simulink model "actuator_control"  (R2016b)
settings: configuration reference "Configuration4khz" (kept outside this file)
values from neighbouring files (symbols this model uses):
  sample_time = 0.0005    [ElmoIncremental.m]
undefined symbols (not defined in the file or in its folder): A_kalman_sea_swing_back, A_kalman_sea_swing_front, A_kalman_swing_load, A_lpf_1to4, A_lpf_dtau, A_lpf_sea_kalman_velocities, B1_lpf_1to4, B1_lpf_dtau, B1_lpf_sea_kalman_velocities, B2_lpf_1to4, B2_lpf_dtau, B2_lpf_sea_kalman_velocities, B_kalman_sea_swing_back, B_kalman_sea_swing_front, B_kalman_swing_load, C_kalman_sea_swing, C_kalman_swing_load, DiscIntNeverNeededParam, Discrete, elmo_sample_time, fdesignblkfcn, gcbh, initial_dx_estimate, j_segments, k_sea_low, kalman_load_to_deflect_transmission, lateral_motor_efficiency, LEG_MTR_GEAR_RATIO, P0_kalman_sea_swing, P0_kalman_swing_load, Q_kalman_load_torque, Q_kalman_rotor_torque, Q_kalman_trunk_torque, R_kalman_absolute_fail, R_kalman_absolute_normal, R_kalman_incremental_loaded, R_kalman_incremental_unloaded, sea_kalman_sample_time, swing_collision_damping_rate, Time
libraries: simulink x17, ctrlSharedLib x8, dsparch4 x5, dspfdesign x1
(part 1 of 3)
settings Model: Creator=wmartin  LastModifiedBy=Will
settings ConfigSetRef: SourceLocation=Base Workspace

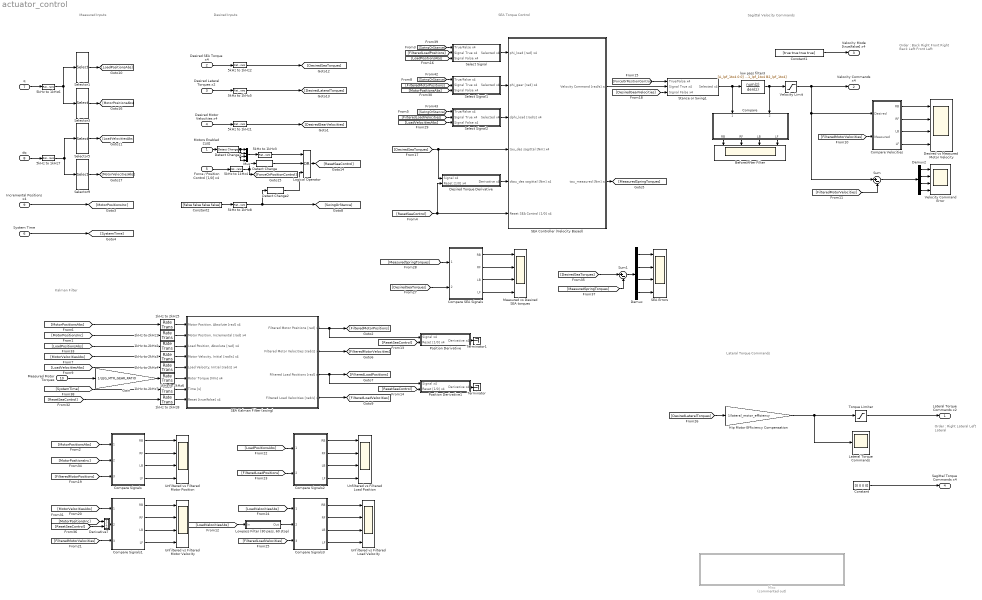
== system actuator_control ==
  note: Order :
      | Back Right
      | Front Right
      | Back Left
      | Front Left
  note: Order :
      | Right Lateral
      | Left Lateral
  note: SEA Torque Control
  note: Lateral Torque Commands
  note: Sagittal Velocity Commands
  note: Measured Inputs
  note: Desired Inputs
  note: Kalman Filter
  Motors Enabled [1/0] : Inport  OutDataTypeStr=boolean  PortDimensions=1  Interpolate=off
  Desired SEA Torque x4 : Inport  Port=2  OutDataTypeStr=double  Unit=N*m  PortDimensions=4  SampleTime=sample_time  Interpolate=off
  Desired Lateral Torques x2 : Inport  Port=3  OutDataTypeStr=double  Unit=N*m  PortDimensions=2  SampleTime=sample_time  Interpolate=off
  Desired Motor Velocities x4 : Inport  Port=4  OutDataTypeStr=double  Unit=rad/sec  PortDimensions=4  SampleTime=sample_time  Interpolate=off
  Force / Position Control [1/0] x4 : Inport  Port=5  OutDataTypeStr=boolean  PortDimensions=4  SampleTime=sample_time  Interpolate=off
  System Time : Inport  Port=6  OutDataTypeStr=double  Unit=sec  PortDimensions=1  Interpolate=off
  q : Inport  Port=7  OutDataTypeStr=double  PortDimensions=13  SampleTime=sample_time  Interpolate=off
  dq : Inport  Port=8  OutDataTypeStr=double  PortDimensions=13  SampleTime=sample_time  Interpolate=off
  Incremental Positions x4 : Inport  Port=9  OutDataTypeStr=double  Unit=rad  PortDimensions=4  Interpolate=off
  Measured Motor Torques : Inport  Port=10  OutDataTypeStr=double  Unit=N*m  PortDimensions=4  Interpolate=off
  1kHz to 2kHz{1..8} (8 alike) : RateTransition  Deterministic=off  OutPortSampleTime=sea_kalman_sample_time
  5kHz to 1kHz{1..8} (8 alike) : RateTransition  Deterministic=off  OutPortSampleTime=elmo_sample_time
  Before/After Filter : Scope  NumInputPorts=4
  Compare : Subsystem
  Compare SEA Signals : Subsystem
  Compare Signals : Subsystem
  Compare Signals1 : Subsystem
  Compare Signals2 : Subsystem
  Compare Signals3 : Subsystem
  Compare Velocities : Subsystem
  Constant : Constant  Value=[0 0 0 0]
  Constant1 : Constant  Value=[true true true true]
  Constant2 : Constant  Value=[false false false false]
  Demux : Demux
  Demux2 : Demux
  Derivative7 : Subsystem
  Desired Torque Derivative : Subsystem
  Desired vs Measured Motor Velocity : Scope  NumInputPorts=4
  Detect Change : simulink/Logic and Bit Operations/Detect Change  vinit=0  InputProcessing=Inherited  OutDataTypeStr=boolean
  Detect Change1 : simulink/Logic and Bit Operations/Detect Change  vinit=0  InputProcessing=Inherited  OutDataTypeStr=boolean
  Detect Change2 : simulink/Logic and Bit Operations/Detect Change  vinit=0  InputProcessing=Inherited  OutDataTypeStr=boolean
  Gain : Gain  Gain=1/LEG_MTR_GEAR_RATIO
  Hip Motor Efficiency Compensation : Gain  Gain=1/lateral_motor_efficiency
  Lateral Torque Commands : Scope
  Logical Operator : Logic  Operator=OR  Inputs=3  AllPortsSameDT=off  OutDataTypeStr=boolean
  "Lowpass Filter (30 pass, 60 stop)" : Subsystem  DialogController=fdesignblkfcn  InitFcn=fdesignblkfcn(gcbh, {'InitFcn'});  mask(Lowpass Filter){}
      mask help: Design a lowpass filter
      settings: CopyFcn=fdesignblkfcn(gcbh, {'CopyFcn'});
      mask Help: helpview(mapfilelocation('dsp'), 'dsplowpassfilter');
      mask Display: disp('Lowpass')
  Measured vs Desired SEA torques : Scope  NumInputPorts=4
  Misc : Subsystem  Commented=on
  Mux : Mux
  Position Derivative : Subsystem
  Position Derivative1 : Subsystem
  SEA Controller (Velocity Based) : Subsystem
  SEA Errors : Scope  NumInputPorts=4
  SEA Kalman Filter (swing) : Subsystem
  Select Signal : Subsystem
  Select Signal1 : Subsystem
  Select Signal2 : Subsystem
  Selector1 : Selector  InputPortWidth=13  IndexOptions=Index vector (dialog)  Indices=[1 3 5 7]  OutputSizes=1
  Selector3 : Selector  InputPortWidth=13  IndexOptions=Index vector (dialog)  Indices=[2 4 6 8]  OutputSizes=1
  Selector5 : Selector  InputPortWidth=13  IndexOptions=Index vector (dialog)  Indices=[1 3 5 7]  OutputSizes=1
  Selector9 : Selector  InputPortWidth=13  IndexOptions=Index vector (dialog)  Indices=[2 4 6 8]  OutputSizes=1
  Stance or Swing1 : Subsystem
  Sum : Sum  Inputs=|+-
  Sum1 : Sum  Inputs=|+-
  Terminator : Terminator
  Terminator1 : Terminator
  Torque Limiter : Saturate  UpperLimit=200  LowerLimit=-200
      settings: AttributesFormatString=Hi: %<UpperLimit>\nLo: %<LowerLimit>
  Unfiltered vs Filtered Load Position : Scope  NumInputPorts=4
  Unfiltered vs Filtered Load Velocity : Scope  NumInputPorts=4
  Unfiltered vs Filtered Motor Position : Scope  NumInputPorts=4
  Unfiltered vs Filtered Motor Velocity : Scope  NumInputPorts=4
  Velocity Command Error : Scope  NumInputPorts=4
  Velocity Limit : Saturate  UpperLimit=6  LowerLimit=-6
      settings: AttributesFormatString=Hi: %<UpperLimit>\nLo: %<LowerLimit>
  low pass filter3 : DiscreteTransferFcn  Numerator=[A_lpf_1to4 0 0]  Denominator=[1 B1_lpf_1to4 B2_lpf_1to4]  SampleTime=elmo_sample_time
  Lateral Torque Commands x2 : Outport  OutDataTypeStr=double  Unit=N*m  PortDimensions=2  InitialOutput=[0 0 0 0 0 0]
  Velocity Commands x4 : Outport  Port=2  Unit=rad/sec  InitialOutput=[0 0 0 0]
  Velocity Mode [true/false] x4 : Outport  Port=3  InitialOutput=[false false false false]
  Sagittal Torque Commands x4 : Outport  Port=4  OutDataTypeStr=double  Unit=N*m  PortDimensions=4  InitialOutput=[0 0 0 0 0 0]
  wires:
  [ForceOrPositionControl] -> Stance or Swing1/1(True/False x4)
  [DesiredGearVelocities] -> Stance or Swing1/3(Signal False x4)
  SEA Kalman Filter (swing)/4(Filtered Load Velocities [rad/s] x4) -> [FilteredLoadVelocities]
  SEA Kalman Filter (swing)/1(Filtered Motor Positions [rad] x4) -> Position Derivative/1(Signal x4), [FilteredMotorPositions]
  1kHz to 2kHz4/1 -> SEA Kalman Filter (swing)/5("Load Velocity, Initial [rad/s] x4")
  1kHz to 2kHz3/1 -> SEA Kalman Filter (swing)/4("Motor Velocity, Initial [rad/s] x4")
  1kHz to 2kHz2/1 -> SEA Kalman Filter (swing)/3("Load Position, Absolute [rad] x4")
  1kHz to 2kHz5/1 -> SEA Kalman Filter (swing)/1("Motor Position, Absolute [rad] x4")
  SEA Controller (Velocity Based)/2(tau_measured [Nm] x4) -> [MeasuredSpringTorques]
  Select Signal/1(Selected x4) -> SEA Controller (Velocity Based)/1(phi_load [rad] x4)
  [DesiredSeaTorques] -> Desired Torque Derivative/1(Signal x4), SEA Controller (Velocity Based)/4(tau_des sagittal [Nm] x4)
  [DesiredLateralTorques] -> Hip Motor Efficiency Compensation/1
  Desired Torque Derivative/1(Derivative x4) -> SEA Controller (Velocity Based)/5(dtau_des sagittal [Nm] x4)
  Hip Motor Efficiency Compensation/1 -> Lateral Torque Commands/1, Torque Limiter/1
  Compare SEA Signals/1(RB) -> Measured vs Desired SEA torques/1
  Compare SEA Signals/2(RF) -> Measured vs Desired SEA torques/2
  Compare SEA Signals/3(LB) -> Measured vs Desired SEA torques/3
  Compare SEA Signals/4(LF) -> Measured vs Desired SEA torques/4
  Compare Velocities/4(LF) -> Desired vs Measured Motor Velocity/4
  Compare Velocities/3(LB) -> Desired vs Measured Motor Velocity/3
  Compare Velocities/1(RB) -> Desired vs Measured Motor Velocity/1
  Compare Velocities/2(RF) -> Desired vs Measured Motor Velocity/2
  [MeasuredSpringTorques] -> Compare SEA Signals/1(1)
  Constant1/1 -> Velocity Mode [true/false] x4/1
  Select Signal1/1(Selected x4) -> SEA Controller (Velocity Based)/2(phi_gear [rad] x4)
  [FilteredMotorVelocities] -> Compare Velocities/2(Measured)
  Demux2/4 -> Velocity Command Error/4
  Demux2/3 -> Velocity Command Error/3
  Demux2/2 -> Velocity Command Error/2
  Demux2/1 -> Velocity Command Error/1
  SEA Controller (Velocity Based)/1(Velocity Command [rad/s] x4) -> Stance or Swing1/2(Signal True x4)
  [MeasuredSpringTorques] -> Sum1/2
  [DesiredSeaTorques] -> Sum1/1
  Demux/1 -> SEA Errors/1
  Demux/4 -> SEA Errors/4
  Demux/3 -> SEA Errors/3
  Demux/2 -> SEA Errors/2
  [LoadPositionsAbs] -> 1kHz to 2kHz2/1
  [MotorPositionsAbs] -> 1kHz to 2kHz5/1
  [MotorPositionsInc] -> 1kHz to 2kHz1/1
  [MotorVelocitiesAbs] -> 1kHz to 2kHz3/1
  [LoadVelocitiesAbs] -> 1kHz to 2kHz4/1
  Selector1/1 -> [LoadPositionsAbs]
  Selector5/1 -> [LoadVelocitiesAbs]
  Force / Position Control [1/0] x4/1 -> 5kHz to 1kHz4/1
  Logical Operator/1 -> [ResetSeaControl]
  Mux/1 -> 5kHz to 1kHz3/1
  Selector3/1 -> [MotorPositionsAbs]
  Detect Change/1 -> Logical Operator/2
  Desired Motor Velocities x4/1 -> 5kHz to 1kHz1/1
  Selector9/1 -> [MotorVelocitiesAbs]
  System Time/1 -> [SystemTime]
  Incremental Positions x4/1 -> [MotorPositionsInc]
  Compare Signals/4(LF) -> Unfiltered vs Filtered Motor Position/4
  Compare Signals/3(LB) -> Unfiltered vs Filtered Motor Position/3
  Compare Signals/2(RF) -> Unfiltered vs Filtered Motor Position/2
  Compare Signals/1(RB) -> Unfiltered vs Filtered Motor Position/1
  [MotorPositionsAbs] -> Compare Signals/1(1)
  [FilteredMotorPositions] -> Compare Signals/3(3)
  Compare Signals1/4(LF) -> Unfiltered vs Filtered Motor Velocity/4
  Compare Signals1/3(LB) -> Unfiltered vs Filtered Motor Velocity/3
  Compare Signals1/2(RF) -> Unfiltered vs Filtered Motor Velocity/2
  Compare Signals1/1(RB) -> Unfiltered vs Filtered Motor Velocity/1
  [MotorVelocitiesAbs] -> Compare Signals1/1(1)
  [FilteredMotorVelocities] -> Compare Signals1/3(3)
  Compare Signals2/4(LF) -> Unfiltered vs Filtered Load Position/4
  Compare Signals2/3(LB) -> Unfiltered vs Filtered Load Position/3
  Compare Signals2/2(RF) -> Unfiltered vs Filtered Load Position/2
  Compare Signals2/1(RB) -> Unfiltered vs Filtered Load Position/1
  [LoadPositionsAbs] -> Compare Signals2/1(1)
  [FilteredLoadPositions] -> Compare Signals2/2(2)
  Compare Signals3/4(LF) -> Unfiltered vs Filtered Load Velocity/4
  Compare Signals3/3(LB) -> Unfiltered vs Filtered Load Velocity/3
  Compare Signals3/2(RF) -> Unfiltered vs Filtered Load Velocity/2
  [LoadVelocitiesAbs] -> Compare Signals3/1(1)
  [FilteredLoadVelocities] -> Compare Signals3/3(3)
  [DesiredSeaTorques] -> Compare SEA Signals/2(2)
  SEA Kalman Filter (swing)/2(Filtered Motor Velocities [rad/s] x4) -> [FilteredMotorVelocities]
  1kHz to 2kHz1/1 -> SEA Kalman Filter (swing)/2("Motor Position, Incremental [rad] x4")
  1kHz to 2kHz6/1 -> SEA Kalman Filter (swing)/6(Rotor Torque [Nm] x4)
  [MotorPositionsInc] -> Compare Signals/2(2)
  Measured Motor Torques/1 -> Gain/1
  Gain/1 -> 1kHz to 2kHz6/1
  [ResetSeaControl] -> Desired Torque Derivative/2(Reset [1/0] x4), SEA Controller (Velocity Based)/6(Reset SEA Control [1/0] x4)
  Derivative7/1(Derivative x4) -> Compare Signals1/2(2)
  [MotorPositionsInc] -> Derivative7/1(Signal x4)
  [ResetSeaControl] -> Derivative7/2(Reset [1/0] x4)
  Sum1/1 -> Demux/1
  Sum/1 -> Demux2/1
  1kHz to 2kHz7/1 -> SEA Kalman Filter (swing)/7(Time [s])
  [SystemTime] -> 1kHz to 2kHz7/1
  Compare Signals3/1(RB) -> Unfiltered vs Filtered Load Velocity/1
  [FilteredMotorVelocities] -> Sum/2
  Velocity Limit/1 -> Sum/1, Compare Velocities/1(Desired), Velocity Commands x4/1
  Desired Lateral Torques x2/1 -> 5kHz to 1kHz5/1
  5kHz to 1kHz1/1 -> [DesiredGearVelocities]
  5kHz to 1kHz3/1 -> Logical Operator/1
  5kHz to 1kHz4/1 -> [ForceOrPositionControl], Detect Change/1
  Torque Limiter/1 -> Lateral Torque Commands x2/1
  "Lowpass Filter (30 pass, 60 stop)"/1(Out) -> Compare Signals3/2(2)
  [LoadVelocitiesAbs] -> "Lowpass Filter (30 pass, 60 stop)"/1(In)
  [ResetSeaControl] -> Position Derivative/2(Reset [1/0] x4)
  SEA Kalman Filter (swing)/3(Filtered Load Positions [rad] x4) -> Position Derivative1/1(Signal x4), [FilteredLoadPositions]
  [ResetSeaControl] -> Position Derivative1/2(Reset [1/0] x4)
  Position Derivative/1(Derivative x4) -> Terminator1/1
  Constant/1 -> Sagittal Torque Commands x4/1
  q/1 -> 5kHz to 1kHz6/1
  dq/1 -> 5kHz to 1kHz7/1
  Motors Enabled [1/0]/1 -> Detect Change1/1
  Detect Change1/1 -> Mux/4, Mux/3, Mux/2, Mux/1
  Position Derivative1/1(Derivative x4) -> Terminator/1
  Select Signal2/1(Selected x4) -> SEA Controller (Velocity Based)/3(dphi_load [rad/s] x4)
  Stance or Swing1/1(Selected x4) -> Compare/1(1), low pass filter3/1
  Compare/4(LF) -> Before/After Filter/4
  Compare/3(LB) -> Before/After Filter/3
  Compare/2(RF) -> Before/After Filter/2
  Compare/1(RB) -> Before/After Filter/1
  5kHz to 1kHz5/1 -> [DesiredLateralTorques]
  5kHz to 1kHz6/1 -> Selector1/1, Selector3/1
  5kHz to 1kHz7/1 -> Selector5/1, Selector9/1
  low pass filter3/1 -> Compare/2(2), Velocity Limit/1
  5kHz to 1kHz8/1 -> Detect Change2/1, [SwingOrStance]
  Detect Change2/1 -> Logical Operator/3
  [SwingOrStance] -> Select Signal/1(True/False x4)
  [FilteredLoadPositions] -> Select Signal/2(Signal True x4)
  [LoadPositionsAbs] -> Select Signal/3(Signal False x4)
  [SwingOrStance] -> Select Signal1/1(True/False x4)
  [SwingOrStance] -> Select Signal2/1(True/False x4)
  [LoadVelocitiesAbs] -> Select Signal2/3(Signal False x4)
  [FilteredLoadVelocities] -> Select Signal2/2(Signal True x4)
  [MotorPositionsAbs] -> Select Signal1/3(Signal False x4)
  [FilteredMotorPositions] -> Select Signal1/2(Signal True x4)
  5kHz to 1kHz2/1 -> [DesiredSeaTorques]
  [ResetSeaControl] -> 1kHz to 2kHz8/1
  1kHz to 2kHz8/1 -> SEA Kalman Filter (swing)/8(Reset [true/false] x4)
  Constant2/1 -> 5kHz to 1kHz8/1
  Desired SEA Torque x4/1 -> 5kHz to 1kHz2/1

== system actuator_control/Compare ==
  1 : Inport
  2 : Inport  Port=2
  Demux : Demux
  Demux1 : Demux
  Mux{6..9} (4 alike) : Mux  Inputs=2
  RB : Outport
  RF : Outport  Port=2
  LB : Outport  Port=3
  LF : Outport  Port=4
  wires:
  Mux9/1 -> LF/1
  Mux8/1 -> LB/1
  Mux7/1 -> RF/1
  Mux6/1 -> RB/1
  Demux/3 -> Mux8/1
  Demux/2 -> Mux7/1
  Demux1/1 -> Mux6/2
  Demux/1 -> Mux6/1
  Demux/4 -> Mux9/1
  Demux1/4 -> Mux9/2
  2/1 -> Demux1/1
  Demux1/2 -> Mux7/2
  1/1 -> Demux/1
  Demux1/3 -> Mux8/2

== system actuator_control/Compare SEA Signals ==
  1 : Inport
  2 : Inport  Port=2
  Demux : Demux
  Demux1 : Demux
  Mux{6..9} (4 alike) : Mux  Inputs=2
  RB : Outport
  RF : Outport  Port=2
  LB : Outport  Port=3
  LF : Outport  Port=4
  wires:
  Demux/3 -> Mux8/1
  Demux/2 -> Mux7/1
  Demux1/1 -> Mux6/2
  Demux/1 -> Mux6/1
  Demux/4 -> Mux9/1
  Demux1/4 -> Mux9/2
  2/1 -> Demux1/1
  Demux1/2 -> Mux7/2
  1/1 -> Demux/1
  Demux1/3 -> Mux8/2
  Mux6/1 -> RB/1
  Mux7/1 -> RF/1
  Mux9/1 -> LF/1
  Mux8/1 -> LB/1

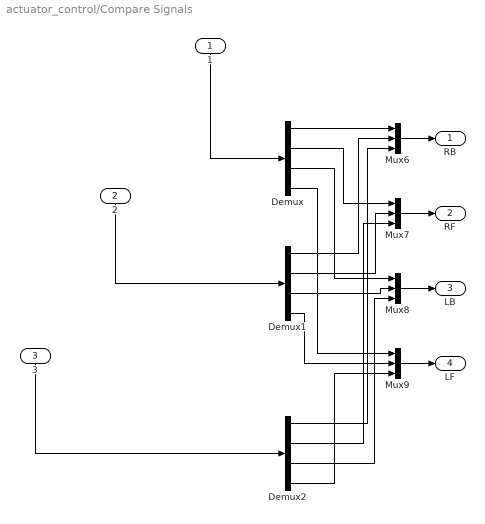
== system actuator_control/Compare Signals ==
  1 : Inport
  2 : Inport  Port=2
  3 : Inport  Port=3
  Demux : Demux
  Demux1 : Demux
  Demux2 : Demux
  Mux{6..9} (4 alike) : Mux  Inputs=3
  RB : Outport
  RF : Outport  Port=2
  LB : Outport  Port=3
  LF : Outport  Port=4
  wires:
  Demux/3 -> Mux8/1
  Demux/2 -> Mux7/1
  Demux1/1 -> Mux6/2
  Demux/1 -> Mux6/1
  Demux/4 -> Mux9/1
  Demux1/4 -> Mux9/2
  2/1 -> Demux1/1
  Demux1/2 -> Mux7/2
  1/1 -> Demux/1
  Demux1/3 -> Mux8/2
  Mux6/1 -> RB/1
  Mux7/1 -> RF/1
  Mux9/1 -> LF/1
  Mux8/1 -> LB/1
  3/1 -> Demux2/1
  Demux2/1 -> Mux6/3
  Demux2/2 -> Mux7/3
  Demux2/3 -> Mux8/3
  Demux2/4 -> Mux9/3

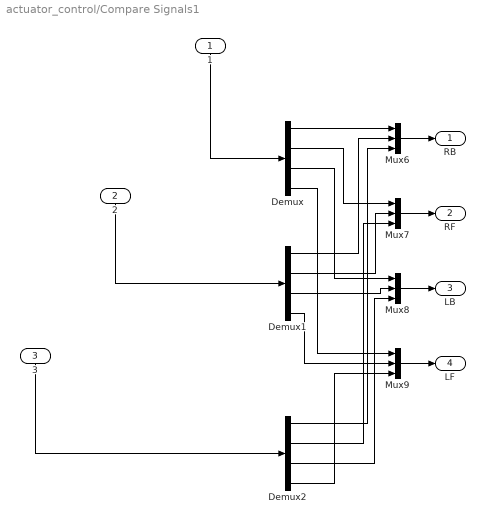
== system actuator_control/Compare Signals1 ==
  1 : Inport
  2 : Inport  Port=2
  3 : Inport  Port=3
  Demux : Demux
  Demux1 : Demux
  Demux2 : Demux
  Mux{6..9} (4 alike) : Mux  Inputs=3
  RB : Outport
  RF : Outport  Port=2
  LB : Outport  Port=3
  LF : Outport  Port=4
  wires:
  Demux2/4 -> Mux9/3
  Demux2/3 -> Mux8/3
  Demux2/2 -> Mux7/3
  Demux2/1 -> Mux6/3
  3/1 -> Demux2/1
  Mux8/1 -> LB/1
  Mux9/1 -> LF/1
  Mux7/1 -> RF/1
  Mux6/1 -> RB/1
  Demux1/3 -> Mux8/2
  1/1 -> Demux/1
  Demux1/2 -> Mux7/2
  2/1 -> Demux1/1
  Demux1/4 -> Mux9/2
  Demux/4 -> Mux9/1
  Demux/1 -> Mux6/1
  Demux1/1 -> Mux6/2
  Demux/2 -> Mux7/1
  Demux/3 -> Mux8/1

== system actuator_control/Compare Signals2 ==
  1 : Inport
  2 : Inport  Port=2
  Demux : Demux
  Demux1 : Demux
  Mux{6..9} (4 alike) : Mux  Inputs=2
  RB : Outport
  RF : Outport  Port=2
  LB : Outport  Port=3
  LF : Outport  Port=4
  wires:
  Demux/3 -> Mux8/1
  Demux/2 -> Mux7/1
  Demux1/1 -> Mux6/2
  Demux/1 -> Mux6/1
  Demux/4 -> Mux9/1
  Demux1/4 -> Mux9/2
  2/1 -> Demux1/1
  Demux1/2 -> Mux7/2
  1/1 -> Demux/1
  Demux1/3 -> Mux8/2
  Mux6/1 -> RB/1
  Mux7/1 -> RF/1
  Mux9/1 -> LF/1
  Mux8/1 -> LB/1

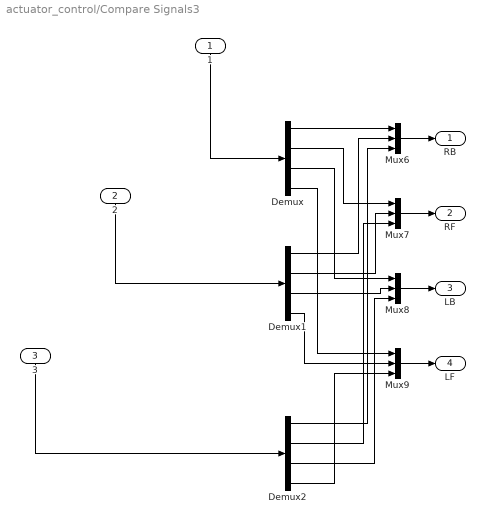
== system actuator_control/Compare Signals3 ==
  1 : Inport
  2 : Inport  Port=2
  3 : Inport  Port=3
  Demux : Demux
  Demux1 : Demux
  Demux2 : Demux
  Mux{6..9} (4 alike) : Mux  Inputs=3
  RB : Outport
  RF : Outport  Port=2
  LB : Outport  Port=3
  LF : Outport  Port=4
  wires:
  Demux2/4 -> Mux9/3
  Demux2/3 -> Mux8/3
  Demux2/2 -> Mux7/3
  Demux2/1 -> Mux6/3
  3/1 -> Demux2/1
  Mux8/1 -> LB/1
  Mux9/1 -> LF/1
  Mux7/1 -> RF/1
  Mux6/1 -> RB/1
  Demux1/3 -> Mux8/2
  1/1 -> Demux/1
  Demux1/2 -> Mux7/2
  2/1 -> Demux1/1
  Demux1/4 -> Mux9/2
  Demux/4 -> Mux9/1
  Demux/1 -> Mux6/1
  Demux1/1 -> Mux6/2
  Demux/2 -> Mux7/1
  Demux/3 -> Mux8/1

== system actuator_control/Compare Velocities ==
  Desired : Inport
  Measured : Inport  Port=2
  Demux : Demux
  Demux1 : Demux
  Mux{6..9} (4 alike) : Mux  Inputs=2
  RB : Outport
  RF : Outport  Port=2
  LB : Outport  Port=3
  LF : Outport  Port=4
  wires:
  Demux1/3 -> Mux8/2
  Desired/1 -> Demux/1
  Demux1/2 -> Mux7/2
  Measured/1 -> Demux1/1
  Demux1/4 -> Mux9/2
  Demux/4 -> Mux9/1
  Demux/1 -> Mux6/1
  Demux1/1 -> Mux6/2
  Demux/2 -> Mux7/1
  Demux/3 -> Mux8/1
  Mux6/1 -> RB/1
  Mux7/1 -> RF/1
  Mux8/1 -> LB/1
  Mux9/1 -> LF/1

== system actuator_control/Derivative7 ==
  Signal x4 : Inport
  Reset [1/0] x4 : Inport  Port=2
  Gain1 : Gain  Gain=1/sea_kalman_sample_time
  Logical Operator : Logic  Operator=NOT  AllPortsSameDT=off  OutDataTypeStr=boolean
  Product : Product
  difference : simulink/Discrete/Difference  ICPrevInput=0.0  InputProcessing=Inherited  OutMin=[]  OutMax=[]  OutDataType=fixdt(1, 16)  OutScaling=2^-10  DoSatur=off
  low pass filter : DiscreteTransferFcn  Numerator=[A_lpf_sea_kalman_velocities 0 0]  Denominator=[1 B1_lpf_sea_kalman_velocities B2_lpf_sea_kalman_velocities]  SampleTime=sea_kalman_sample_time
  Derivative x4 : Outport
  wires:
  Gain1/1 -> difference/1
  Signal x4/1 -> Gain1/1
  difference/1 -> Product/1
  Reset [1/0] x4/1 -> Logical Operator/1
  Logical Operator/1 -> Product/2
  Product/1 -> low pass filter/1
  low pass filter/1 -> Derivative x4/1

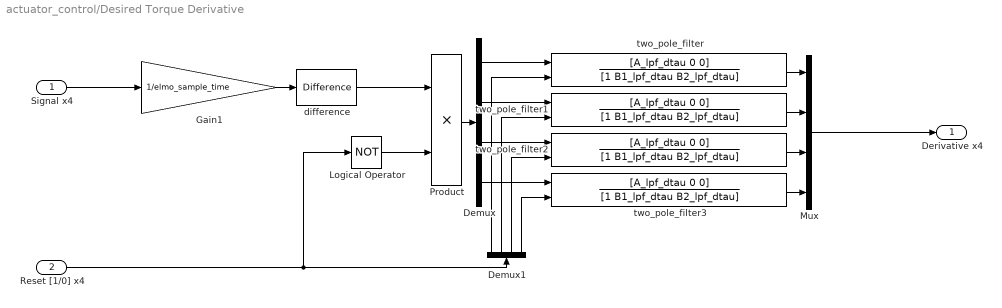
== system actuator_control/Desired Torque Derivative ==
  Signal x4 : Inport
  Reset [1/0] x4 : Inport  Port=2
  Demux : Demux
  Demux1 : Demux
  Gain1 : Gain  Gain=1/elmo_sample_time
  Logical Operator : Logic  Operator=NOT  AllPortsSameDT=off  OutDataTypeStr=boolean
  Mux : Mux
  Product : Product
  difference : simulink/Discrete/Difference  ICPrevInput=0.0  InputProcessing=Inherited  OutMin=[]  OutMax=[]  OutDataType=fixdt(1, 16)  OutScaling=2^-10  DoSatur=off
  two_pole_filter{,1..3} (4 alike) : DiscreteTransferFcn  Numerator=[A_lpf_dtau 0 0]  Denominator=[1 B1_lpf_dtau B2_lpf_dtau]  ExternalReset=Rising  SampleTime=elmo_sample_time
      settings: InputPortMap=u0,r7
  Derivative x4 : Outport
  wires:
  Demux/1 -> two_pole_filter/1
  difference/1 -> Product/1
  Logical Operator/1 -> Product/2
  two_pole_filter/1 -> Mux/1
  Product/1 -> Demux/1
  two_pole_filter1/1 -> Mux/2
  two_pole_filter2/1 -> Mux/3
  two_pole_filter3/1 -> Mux/4
  Demux/2 -> two_pole_filter1/1
  Demux/3 -> two_pole_filter2/1
  Demux/4 -> two_pole_filter3/1
  Demux1/1 -> two_pole_filter/2
  Demux1/2 -> two_pole_filter1/2
  Demux1/3 -> two_pole_filter2/2
  Demux1/4 -> two_pole_filter3/2
  Gain1/1 -> difference/1
  Mux/1 -> Derivative x4/1
  Reset [1/0] x4/1 -> Demux1/1, Logical Operator/1
  Signal x4/1 -> Gain1/1

== system actuator_control/Lowpass Filter (30 pass, 60 stop) ==
  In : Inport
  Generated Filter Block : DiscreteFir  Tag=BlockMethodSubSystem  Coefficients=[-0.04990855361244094 -0.0010461181532544423 -0.0010107744805273023 -0.00095218248250663988 -0.00085849397163504759 -0.00074175367502442866 -0.00058718772776830946 -0.00041184474721322643 -0.00019652887760975509 4.1532722907783075e-05 0.00031999675256174498 0.00061963547362796486 0.00095907702319196237 0.0013114899691414792 0.0017077848126334939 0.0021254626826913022 0.0025760447586962117 0.0030487109199885914 0.0035497166866013206 0.0040832493046027646 0.0046307261794588678 0.0051947242056444003 0.0057923012727255181 0.0063989592738492437 0.0070358610723892474 0.0076729710874219904 0.0083378124160072738 0.0089921015506421835 0.0096759335261809524 0.010331908705729947 0.011024573190749414 0.011633575605025979 0.012404292046454947 0.013110276864067787 0.013752343250190606 0.01444307115793151 0.015092411392359124 0.015755931236486116 0.01638320562971788 0.017012416656076532 0.017610586760412175 0.018198786428169338 0.018753273958556273 0.019289760931779823 0.01978959816621716 0.020267409454217542 0.020714123209904678 0.02112524451621629 0.021506539266400629 0.021843487024455384 0.022166915431959651 0.022425498521847217 0.02263611511837274 0.022838689821158754 0.022982920388946775 0.023100208768407095 0.023159386359289921 0.023188270363550461 0.023159386359289921 0.023100208768407095 0.022982920388946775 0.022838689821158754 0.02263611511837274 0.022425498521847217 0.022166915431959651 0.021843487024455384 0.021506539266400629 0.02112524451621629 0.020714123209904678 0.020267409454217542 0.01978959816621716 0.019289760931779823 0.018753273958556273 0.018198786428169338 0.017610586760412175 0.017012416656076532 0.01638320562971788 0.015755931236486116 0.015092411392359124 0.01444307115793151 0.013752343250190606 0.013110276864067787 0.012404292046454947 0.011633575605025979 0.011024573190749414 0.010331908705729947 0.0096759335261809524 0.0089921015506421835 0.0083378124160072738 0.0076729710874219904 0.0070358610723892474 0.0063989592738492437 0.0057923012727255181 0.0051947242056444003 0.0046307261794588678 0.0040832493046027646 0.0035497166866013206 0.0030487109199885914 0.0025760447586962117 0.0021254626826913022 0.0017077848126334939 0.0013114899691414792 0.00095907702319196237 0.00061963547362796486 0.00031999675256174498 4.1532722907783075e-05 -0.00019652887760975509 -0.00041184474721322643 -0.00058718772776830946 -0.00074175367502442866 -0.00085849397163504759 -0.00095218248250663988 -0.0010107744805273023 -0.0010461181532544423 -0.04990855361244094]
  Out : Outport
  wires:
  In/1 -> Generated Filter Block/1
  Generated Filter Block/1 -> Out/1

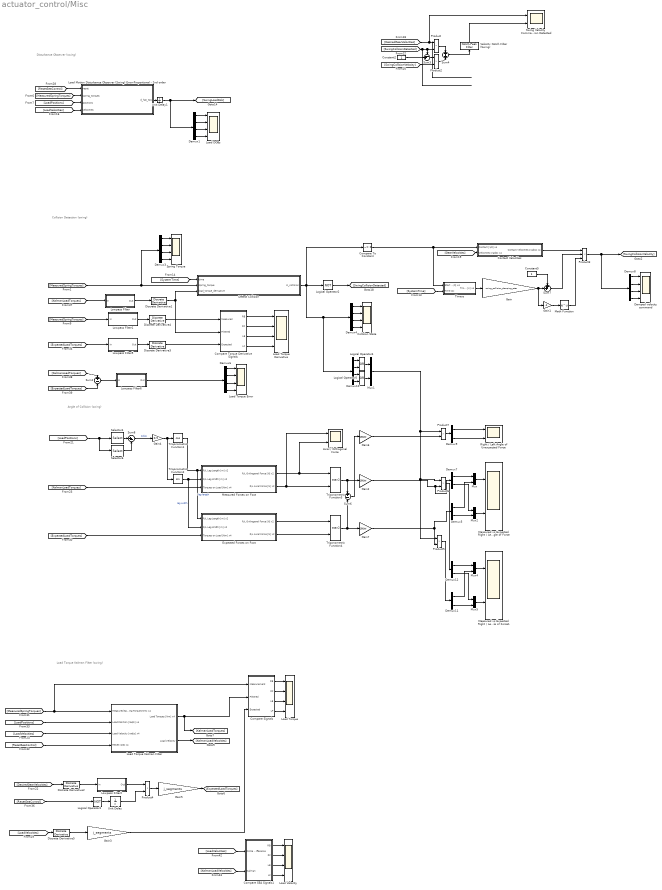
== system actuator_control/Misc ==
  note: Disturbance Observer (swing)
  note: Collision Detection (swing)
  note: Angle of Collision (swing)
  note: Load Torque Kalman Filter (swing)
  Axial / Orthogonal Force : Scope  NumInputPorts=2
  Collision State : Scope  NumInputPorts=4
  Compare To Constant : simulink/Logic and Bit Operations/Compare To Constant  relop=~=  const=0  OutDataTypeStr=boolean
  Compare SEA Signals1 : Subsystem
  Compare Signals : Subsystem
  Compare Torque Derivative Signals : Subsystem
  Constant2 : Constant
  Constant5 : Constant
  Contact Velocities : Subsystem
  Damped velocity command : Scope  NumInputPorts=4
  Demux{1,3..4,6,8,10} (6 alike) : Demux
  Demux{5,7,9,11..12} (5 alike) : Demux  Outputs=2
  Detect Collision : MATLAB Function  TreatAsAtomicUnit=on
  Discrete Derivative{1..5} (5 alike) : simulink/Discrete/Discrete Derivative  gainval=1.0  ICPrevScaledInput=0.0  OutMin=[]  OutMax=[]  OutDataType=fixdt(1, 16)  OutScaling=2^-10  DoSatur=off
  Expected Forces on Foot : Subsystem
  Gain : Gain  Gain=swing_collision_damping_rate
  Gain1 : Gain  Gain=-1
  Gain2 : Gain  Gain=180/pi
  Gain3 : Gain  Gain=j_segments
  Gain4 : Gain  Gain=0.5
  Gain5 : Gain  Gain=j_segments
  Gain6 : Gain  Gain=180/pi
  Gain7 : Gain  Gain=180/pi
  Load DOBs : Scope  NumInputPorts=4
  Load Motion Disturbance Observer (Swing) Error-Proportional - 2nd order : MATLAB Function  TreatAsAtomicUnit=on
  Load Torque : Scope  NumInputPorts=4
  Load Torque Derivative : Scope  NumInputPorts=4
  Load Torque Error : Scope  NumInputPorts=4
  Load Torque Kalman Filter : Subsystem
  Load Velocity : Scope  NumInputPorts=4
  Logical Operator2 : Logic  Operator=NOT  AllPortsSameDT=off  OutDataTypeStr=boolean
  Logical Operator3 : Logic  Operator=NOT  AllPortsSameDT=off  OutDataTypeStr=boolean
  Logical Operator4 : Logic  Operator=OR  AllPortsSameDT=off  OutDataTypeStr=boolean
  Logical Operator5 : Logic  Operator=OR  AllPortsSameDT=off  OutDataTypeStr=boolean
  Lowpass Filter : Subsystem  DialogController=fdesignblkfcn  InitFcn=fdesignblkfcn(gcbh, {'InitFcn'});  mask(Lowpass Filter){}
      mask help: Design a lowpass filter
      settings: CopyFcn=fdesignblkfcn(gcbh, {'CopyFcn'});
      mask Help: helpview(mapfilelocation('dsp'), 'dsplowpassfilter');
      mask Display: disp('Lowpass')
  Lowpass Filter1 : Subsystem  DialogController=fdesignblkfcn  InitFcn=fdesignblkfcn(gcbh, {'InitFcn'});  mask(Lowpass Filter){}
      mask help: Design a lowpass filter
      settings: CopyFcn=fdesignblkfcn(gcbh, {'CopyFcn'});
      mask Help: helpview(mapfilelocation('dsp'), 'dsplowpassfilter');
      mask Display: disp('Lowpass')
  Lowpass Filter2 : Subsystem  DialogController=fdesignblkfcn  InitFcn=fdesignblkfcn(gcbh, {'InitFcn'});  mask(Lowpass Filter){}
      mask help: Design a lowpass filter
      settings: CopyFcn=fdesignblkfcn(gcbh, {'CopyFcn'});
      mask Help: helpview(mapfilelocation('dsp'), 'dsplowpassfilter');
      mask Display: disp('Lowpass')
  Lowpass Filter5 : Subsystem  DialogController=fdesignblkfcn  InitFcn=fdesignblkfcn(gcbh, {'InitFcn'});  mask(Lowpass Filter){}
      mask help: Design a lowpass filter
      settings: CopyFcn=fdesignblkfcn(gcbh, {'CopyFcn'});
      mask Help: helpview(mapfilelocation('dsp'), 'dsplowpassfilter');
      mask Display: disp('Lowpass')
  Lowpass Filter6 : Subsystem  DialogController=fdesignblkfcn  InitFcn=fdesignblkfcn(gcbh, {'InitFcn'});  mask(Lowpass Filter){}
      mask help: Design a lowpass filter
      settings: CopyFcn=fdesignblkfcn(gcbh, {'CopyFcn'});
      mask Help: helpview(mapfilelocation('dsp'), 'dsplowpassfilter');
      mask Display: disp('Lowpass')
  Math Function : Math  SaturateOnIntegerOverflow=on
  Measured Forces on Foot : Subsystem
  Measured vs Expected Right / Left Angle of Force : Scope  NumInputPorts=2
  Measured vs Expected Right / Left Angle of Force1 : Scope  NumInputPorts=2
  Mux{,1..2,4..5} (5 alike) : Mux  Inputs=2
  Product{,2,4..7} (6 alike) : Product
  Product3 : Product  Inputs=3
  Right / Left Angle of Unexpected Force : Scope  NumInputPorts=2
  Selector4 : Selector  InputPortWidth=4  IndexOptions=Index vector (dialog)  Indices=[1 3]  OutputSizes=1
  Selector6 : Selector  InputPortWidth=4  IndexOptions=Index vector (dialog)  Indices=[2 4]  OutputSizes=1
  Spring Torque : Scope  NumInputPorts=4
  Sum2 : Sum  Inputs=+|-
  Sum3 : Sum  Inputs=-+|
  Sum4 : Sum  Inputs=+|+
  Sum6 : Sum  Inputs=+|-
  Sum7 : Sum  Inputs=++|
  Sum8 : Sum  Inputs=|+-
  Swing Velocity Commands Collision Detected : Scope  NumInputPorts=2
  Timers : Subsystem
  Trigonometric Function1 : Trigonometry  Operator=cos
  Trigonometric Function2 : Trigonometry
  Trigonometric Function3 : Trigonometry  Operator=atan2
  Trigonometric Function4 : Trigonometry  Operator=atan2
  Unit Delay : UnitDelay  SampleTime=-1
  Unit Delay1 : UnitDelay  SampleTime=sample_time
  Velocity Notch Filter (Swing) : dspfdesign/Notch-Peak Filter  Specification=Quality factor and center frequency  Bandwidth=27  QualityFactor=2.5  CenterFrequency=27  BandwidthCoefficient=0.72654  CenterFrequencyCoefficient=0  Output=Notch  InheritSampleRate=off  SampleRate=update_freq  SimulateUsing=Code generation
  wires:
  Load Motion Disturbance Observer (Swing) Error-Proportional - 2nd order/1(d_hat_tp1) -> Unit Delay1/1
  [MeasuredSpringTorques] -> Load Motion Disturbance Observer (Swing) Error-Proportional - 2nd order/2(spring_torques)
  [LoadVelocities] -> Load Motion Disturbance Observer (Swing) Error-Proportional - 2nd order/4(velocities)
  [ResetSeaControl] -> Load Motion Disturbance Observer (Swing) Error-Proportional - 2nd order/1(reset)
  [LoadPositions] -> Load Motion Disturbance Observer (Swing) Error-Proportional - 2nd order/3(positions)
  Demux1/1 -> Load DOBs/1
  Unit Delay1/1 -> [SwingLoadDob], Demux1/1
  Demux1/2 -> Load DOBs/2
  Demux1/3 -> Load DOBs/3
  Demux1/4 -> Load DOBs/4
  [SwingCollisionDetected] -> Product/2, Sum3/1
  Constant2/1 -> Sum3/2
  Product/1 -> Sum4/1
  Product2/1 -> Sum4/2
  Sum3/1 -> Product2/1
  [DesiredGearVelocities] -> Swing Velocity Commands Collision Detected/1, Product/1
  Sum4/1 -> Velocity Notch Filter (Swing)/1
  [SwingCollisionVelocity] -> Product2/2
  Demux3/4 -> Spring Torque/4
  Demux3/3 -> Spring Torque/3
  Demux3/2 -> Spring Torque/2
  Demux3/1 -> Spring Torque/1
  [KalmanLoadTorques] -> Lowpass Filter/1(In)
  Detect Collision/1(in_collision) -> Compare To Constant/1, Demux10/1, Demux4/1, Logical Operator2/1
  [GearVelocities] -> Contact Velocities/2(Velocities [rad/s] x4)
  Contact Velocities/1(Contact Velocities [rad/s] x4) -> Product3/1
  Compare To Constant/1 -> Contact Velocities/1(Contact [1/0] x4), Timers/1(Start [1/0] x4)
  Timers/1(Timer [s] x4) -> Gain/1
  Gain/1 -> Gain1/1, Sum7/2
  Constant5/1 -> Sum7/1
  Gain1/1 -> Math Function/1
  Math Function/1 -> Product3/3
  Product3/1 -> [SwingCollisionVelocity], Demux8/1
  Demux8/3 -> Damped velocity command/3
  Demux8/2 -> Damped velocity command/2
  Demux8/1 -> Damped velocity command/1
  Demux8/4 -> Damped velocity command/4
  [SystemTime] -> Timers/2(Time [s])
  [SystemTime] -> Detect Collision/1(time)
  Demux4/3 -> Collision State/3
  Demux4/2 -> Collision State/2
  Demux4/1 -> Collision State/1
  Demux4/4 -> Collision State/4
  Logical Operator2/1 -> [SwingCollisionDetected]
  Selector4/1 -> Sum8/1
  Sum8/1 -> Gain4/1  "splay"
  Gain4/1 -> Trigonometric Function2/1, Trigonometric Function1/1
  [LoadPositions] -> Selector6/1, Selector4/1
  Demux7/2 -> Mux2/1
  Demux7/1 -> Mux/1
  Trigonometric Function3/1 -> Sum6/1, Gain2/1
  [ExpectedLoadTorques] -> Lowpass Filter5/1(In)
  Lowpass Filter5/1(Out) -> Discrete Derivative3/1
  Compare Torque Derivative Signals/4(LF) -> Load Torque Derivative/4
  Compare Torque Derivative Signals/3(LB) -> Load Torque Derivative/3
  Compare Torque Derivative Signals/2(RF) -> Load Torque Derivative/2
  Compare Torque Derivative Signals/1(RB) -> Load Torque Derivative/1
  [MeasuredSpringTorques] -> Lowpass Filter1/1(In)
  Lowpass Filter1/1(Out) -> Discrete Derivative4/1
  Discrete Derivative4/1 -> Compare Torque Derivative Signals/1(Measured)
  Demux6/3 -> Load Torque Error/3
  Demux6/2 -> Load Torque Error/2
  Demux6/1 -> Load Torque Error/1
  Demux6/4 -> Load Torque Error/4
  [KalmanLoadTorques] -> Sum2/1
  [ExpectedLoadTorques] -> Sum2/2
  Sum2/1 -> Lowpass Filter6/1(In)
  Discrete Derivative3/1 -> Compare Torque Derivative Signals/3(Expected)
  Selector6/1 -> Sum8/2
  Demux5/2 -> Mux2/2
  Demux5/1 -> Mux/2
  Demux10/1 -> Logical Operator4/1
  Demux10/2 -> Logical Operator4/2
  Demux10/4 -> Logical Operator5/2
  Demux10/3 -> Logical Operator5/1
  Logical Operator4/1 -> Mux1/1
  Logical Operator5/1 -> Mux1/2
  Sum7/1 -> Product3/2
  Discrete Derivative1/1 -> Compare Torque Derivative Signals/2(Filtered), Detect Collision/3(load_torque_derivative)
  Lowpass Filter6/1(Out) -> Demux6/1
  Lowpass Filter/1(Out) -> Discrete Derivative1/1
  Trigonometric Function1/1 -> Expected Forces on Foot/1(R/L Leg Length [m] x2), Measured Forces on Foot/1(R/L Leg Length [m] x2)  "leg length"
  Trigonometric Function2/1 -> Measured Forces on Foot/2(R/L Leg Width [m] x2), Expected Forces on Foot/2(R/L Leg Width [m] x2)  "leg width"
  [KalmanLoadTorques] -> Measured Forces on Foot/3(Torques on Load [Nm] x4)
  Measured Forces on Foot/1(R/L Orthogonal Force [N] x2) -> Trigonometric Function3/1, Axial / Orthogonal Force/2
  Measured Forces on Foot/2(R/L Axial Force [N] x2) -> Axial / Orthogonal Force/1, Trigonometric Function3/2
  [ExpectedLoadTorques] -> Expected Forces on Foot/3(Torques on Load [Nm] x4)
  Expected Forces on Foot/1(R/L Orthogonal Force [N] x2) -> Trigonometric Function4/1
  Trigonometric Function4/1 -> Sum6/2, Gain7/1
  Gain6/1 -> Product7/2
  Demux9/1 -> Right / Left Angle of Unexpected Force/1
  Demux9/2 -> Right / Left Angle of Unexpected Force/2
  Expected Forces on Foot/2(R/L Axial Force [N] x2) -> Trigonometric Function4/2
  Mux2/1 -> Measured vs Expected Right / Left Angle of Force/2
  Mux/1 -> Measured vs Expected Right / Left Angle of Force/1
  Gain7/1 -> Demux5/1, Product5/2
  Gain2/1 -> Demux7/1, Product6/2
  Mux1/1 -> Product7/1, Product5/1, Product6/1
  Sum6/1 -> Gain6/1
  Product7/1 -> Demux9/1
  Demux12/2 -> Mux5/1
  Demux12/1 -> Mux4/1
  Demux11/2 -> Mux5/2
  Demux11/1 -> Mux4/2
  Mux5/1 -> Measured vs Expected Right / Left Angle of Force1/2
  Mux4/1 -> Measured vs Expected Right / Left Angle of Force1/1
  Product6/1 -> Demux12/1
  Product5/1 -> Demux11/1
  [MeasuredSpringTorques] -> Demux3/1, Detect Collision/2(spring_torque)
  [LoadVelocities] -> Load Torque Kalman Filter/3(Load Velocity [rad/s] x4)
  [ResetSeaControl] -> Load Torque Kalman Filter/4(Reset [1/0] x4)
  Compare Signals/3(LB) -> Load Torque/3
  Compare Signals/2(RF) -> Load Torque/2
  Compare Signals/4(LF) -> Load Torque/4
  Compare Signals/1(RB) -> Load Torque/1
  Load Torque Kalman Filter/1(Load Torques [Nm] x4) -> [KalmanLoadTorques], Compare Signals/2(Filtered)
  [MeasuredSpringTorques] -> Compare Signals/1(Measurement), Load Torque Kalman Filter/1(Measured Spring Torque [Nm] x4)
  [LoadPositions] -> Load Torque Kalman Filter/2(Load Position [rad/s] x4)
  Product4/1 -> Gain5/1
  Gain5/1 -> [ExpectedLoadTorques]
  Discrete Derivative2/1 -> Lowpass Filter2/1(In)
  Logical Operator3/1 -> Unit Delay/1
  [ResetSeaControl] -> Logical Operator3/1
  Unit Delay/1 -> Product4/2
  [DesiredGearVelocities] -> Discrete Derivative2/1
  Lowpass Filter2/1(Out) -> Product4/1
  [LoadVelocities] -> Discrete Derivative5/1
  Discrete Derivative5/1 -> Gain3/1
  Gain3/1 -> Compare Signals/3(Expected)
  Load Torque Kalman Filter/2(Load Velocity) -> [KalmanLoadVelocities]
  Compare SEA Signals1/4(LF) -> Load Velocity/4
  Compare SEA Signals1/3(LB) -> Load Velocity/3
  Compare SEA Signals1/2(RF) -> Load Velocity/2
  Compare SEA Signals1/1(RB) -> Load Velocity/1
  [KalmanLoadVelocities] -> Compare SEA Signals1/2(Kalman)
  [LoadVelocities] -> Compare SEA Signals1/1(Finite Difference)
  Velocity Notch Filter (Swing)/1 -> Swing Velocity Commands Collision Detected/2

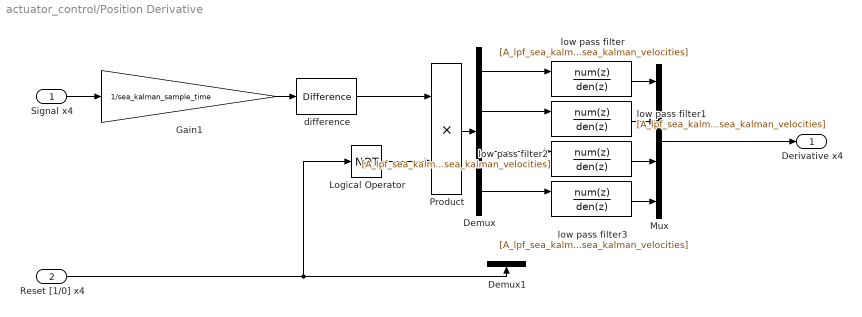
== system actuator_control/Position Derivative ==
  Signal x4 : Inport
  Reset [1/0] x4 : Inport  Port=2
  Demux : Demux
  Demux1 : Demux
  Gain1 : Gain  Gain=1/sea_kalman_sample_time
  Logical Operator : Logic  Operator=NOT  AllPortsSameDT=off  OutDataTypeStr=boolean
  Mux : Mux
  Product : Product
  difference : simulink/Discrete/Difference  ICPrevInput=0.0  InputProcessing=Inherited  OutMin=[]  OutMax=[]  OutDataType=fixdt(1, 16)  OutScaling=2^-10  DoSatur=off
  low pass filter{,1..3} (4 alike) : DiscreteTransferFcn  Numerator=[A_lpf_sea_kalman_velocities 0 0]  Denominator=[1 B1_lpf_sea_kalman_velocities B2_lpf_sea_kalman_velocities]  ExternalReset=Rising  SampleTime=sea_kalman_sample_time
      settings: InputPortMap=u0,r7
  Derivative x4 : Outport
  wires:
  Signal x4/1 -> Gain1/1
  Reset [1/0] x4/1 -> Logical Operator/1, Demux1/1
  Product/1 -> Demux/1
  Gain1/1 -> difference/1
  Demux/4 -> low pass filter3/1
  Demux/3 -> low pass filter2/1
  Demux/2 -> low pass filter1/1
  low pass filter3/1 -> Mux/4
  low pass filter2/1 -> Mux/3
  low pass filter1/1 -> Mux/2
  low pass filter/1 -> Mux/1
  Logical Operator/1 -> Product/2
  difference/1 -> Product/1
  Demux/1 -> low pass filter/1
  Mux/1 -> Derivative x4/1

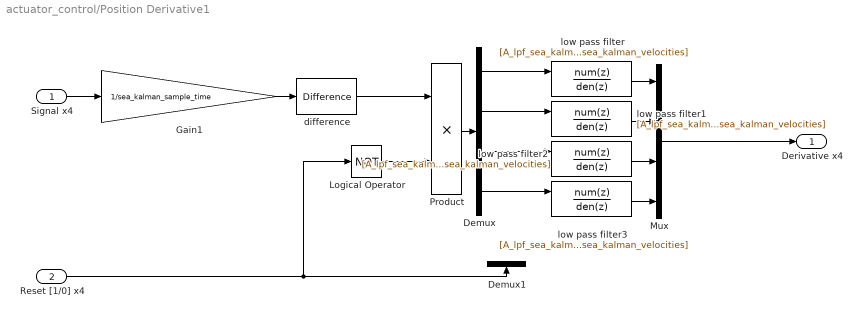
== system actuator_control/Position Derivative1 ==
  Signal x4 : Inport
  Reset [1/0] x4 : Inport  Port=2
  Demux : Demux
  Demux1 : Demux
  Gain1 : Gain  Gain=1/sea_kalman_sample_time
  Logical Operator : Logic  Operator=NOT  AllPortsSameDT=off  OutDataTypeStr=boolean
  Mux : Mux
  Product : Product
  difference : simulink/Discrete/Difference  ICPrevInput=0.0  InputProcessing=Inherited  OutMin=[]  OutMax=[]  OutDataType=fixdt(1, 16)  OutScaling=2^-10  DoSatur=off
  low pass filter{,1..3} (4 alike) : DiscreteTransferFcn  Numerator=[A_lpf_sea_kalman_velocities 0 0]  Denominator=[1 B1_lpf_sea_kalman_velocities B2_lpf_sea_kalman_velocities]  ExternalReset=Rising  SampleTime=sea_kalman_sample_time
      settings: InputPortMap=u0,r7
  Derivative x4 : Outport
  wires:
  Demux/1 -> low pass filter/1
  difference/1 -> Product/1
  Logical Operator/1 -> Product/2
  low pass filter/1 -> Mux/1
  low pass filter1/1 -> Mux/2
  low pass filter2/1 -> Mux/3
  low pass filter3/1 -> Mux/4
  Demux/2 -> low pass filter1/1
  Demux/3 -> low pass filter2/1
  Demux/4 -> low pass filter3/1
  Gain1/1 -> difference/1
  Reset [1/0] x4/1 -> Demux1/1, Logical Operator/1
  Signal x4/1 -> Gain1/1
  Mux/1 -> Derivative x4/1
  Product/1 -> Demux/1

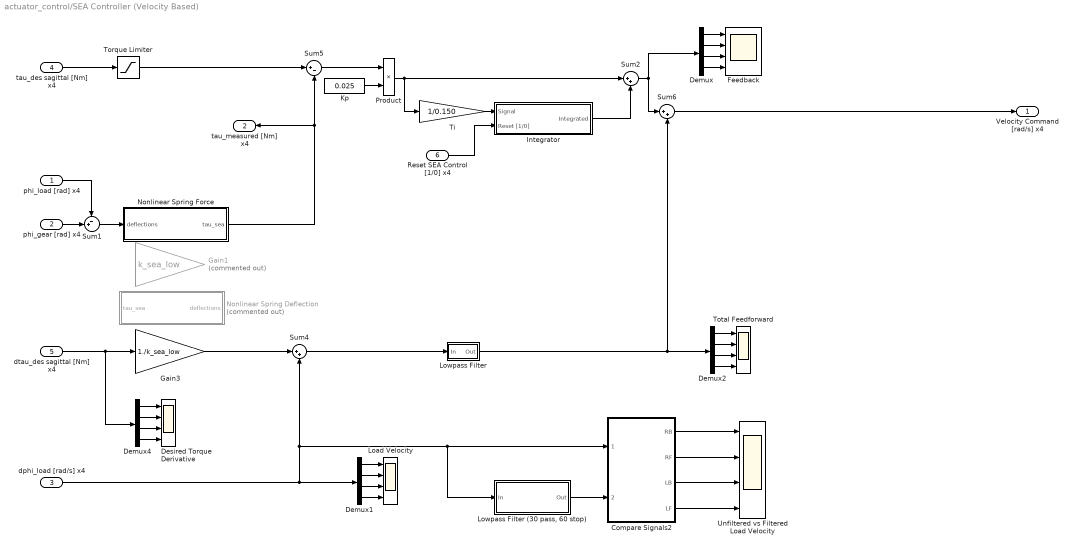
== system actuator_control/SEA Controller (Velocity Based) ==
  phi_load [rad] x4 : Inport
  phi_gear [rad] x4 : Inport  Port=2
  dphi_load [rad/s] x4 : Inport  Port=3
  tau_des sagittal [Nm] x4 : Inport  Port=4
  dtau_des sagittal [Nm] x4 : Inport  Port=5
  Reset SEA Control [1/0] x4 : Inport  Port=6
  Compare Signals2 : Subsystem
  Demux{,1..2,4} (4 alike) : Demux
  Desired Torque Derivative : Scope  NumInputPorts=4
  Feedback : Scope  NumInputPorts=4
  Gain1 : Gain  Commented=on  Gain=k_sea_low
  Gain3 : Gain  Gain=1./k_sea_low
  Integrator : Subsystem
  Kp : Constant  Value=0.025
  Load Velocity : Scope  NumInputPorts=4
  Lowpass Filter : Subsystem  DialogController=fdesignblkfcn  InitFcn=fdesignblkfcn(gcbh, {'InitFcn'});  mask(Lowpass Filter){}
      mask help: Design a lowpass filter
      settings: CopyFcn=fdesignblkfcn(gcbh, {'CopyFcn'});
      mask Help: helpview(mapfilelocation('dsp'), 'dsplowpassfilter');
      mask Display: disp('Lowpass')
  "Lowpass Filter (30 pass, 60 stop)" : Subsystem  DialogController=fdesignblkfcn  InitFcn=fdesignblkfcn(gcbh, {'InitFcn'});  mask(Lowpass Filter){}
      mask help: Design a lowpass filter
      settings: CopyFcn=fdesignblkfcn(gcbh, {'CopyFcn'});
      mask Help: helpview(mapfilelocation('dsp'), 'dsplowpassfilter');
      mask Display: disp('Lowpass')
  Nonlinear Spring Deflection : MATLAB Function  Commented=on  TreatAsAtomicUnit=on
  Nonlinear Spring Force : MATLAB Function  TreatAsAtomicUnit=on
  Product : Product
  Sum1 : Sum  Inputs=-+|
  Sum2 : Sum  Inputs=|++
  Sum4 : Sum  Inputs=|++
  Sum5 : Sum  Inputs=|+-
  Sum6 : Sum  Inputs=|++
  Ti : Gain  Gain=1/0.150
  Torque Limiter : Saturate  UpperLimit=900  LowerLimit=-900
      settings: AttributesFormatString=Hi: %<UpperLimit>\nLo: %<LowerLimit>
  Total Feedforward : Scope  NumInputPorts=4
  Unfiltered vs Filtered Load Velocity : Scope  NumInputPorts=4
  Velocity Command [rad/s] x4 : Outport  PortDimensions=4
  tau_measured [Nm] x4 : Outport  Port=2
  wires:
  Demux1/4 -> Load Velocity/4
  Demux2/4 -> Total Feedforward/4
  Demux2/3 -> Total Feedforward/3
  Demux2/2 -> Total Feedforward/2
  Demux2/1 -> Total Feedforward/1
  Demux1/3 -> Load Velocity/3
  Demux1/2 -> Load Velocity/2
  Demux1/1 -> Load Velocity/1
  Sum1/1 -> Nonlinear Spring Force/1(deflections)
  Nonlinear Spring Force/1(tau_sea) -> tau_measured [Nm] x4/1, Sum5/2
  Gain3/1 -> Sum4/1
  dtau_des sagittal [Nm] x4/1 -> Demux4/1, Gain3/1
  Sum5/1 -> Product/1
  Kp/1 -> Product/2
  Torque Limiter/1 -> Sum5/1
  Demux/4 -> Feedback/4
  Demux/3 -> Feedback/3
  Demux/2 -> Feedback/2
  Demux/1 -> Feedback/1
  tau_des sagittal [Nm] x4/1 -> Torque Limiter/1
  phi_gear [rad] x4/1 -> Sum1/2
  phi_load [rad] x4/1 -> Sum1/1
  Demux4/4 -> Desired Torque Derivative/4
  Demux4/3 -> Desired Torque Derivative/3
  Demux4/2 -> Desired Torque Derivative/2
  Demux4/1 -> Desired Torque Derivative/1
  Product/1 -> Ti/1, Sum2/1
  Sum6/1 -> Velocity Command [rad/s] x4/1
  Ti/1 -> Integrator/1(Signal)
  Reset SEA Control [1/0] x4/1 -> Integrator/2(Reset [1/0])
  Sum2/1 -> Demux/1, Sum6/1
  Integrator/1(Integrated) -> Sum2/2
  Compare Signals2/4(LF) -> Unfiltered vs Filtered Load Velocity/4
  Compare Signals2/3(LB) -> Unfiltered vs Filtered Load Velocity/3
  Compare Signals2/2(RF) -> Unfiltered vs Filtered Load Velocity/2
  Compare Signals2/1(RB) -> Unfiltered vs Filtered Load Velocity/1
  "Lowpass Filter (30 pass, 60 stop)"/1(Out) -> Compare Signals2/2(2)
  dphi_load [rad/s] x4/1 -> "Lowpass Filter (30 pass, 60 stop)"/1(In), Compare Signals2/1(1), Sum4/2, Demux1/1
  Sum4/1 -> Lowpass Filter/1(In)
  Lowpass Filter/1(Out) -> Sum6/2, Demux2/1
